simulink model "final_4"  (Simulink 7.3)
(part 2 of 2)

      |       Name		      "PQ2"
      |       Ports		      [2, 1]
      |       Position		      [1580, 1176, 1605, 1209]
      |       NamePlacement	      "alternate"
      |       DialogController	      "POWERSYS.PowerSysDialog"
      |       FontName		      "Verdana"
      |       FontSize		      11
      |       SourceBlock	      "powerlib_extras/Measurements/3-phase \nInstantaneous \nActive & Reactive Power"
      |       SourceType	      "3-phase instantaneous active and reactive power"
      |       ShowPortLabels	      "FromPortIcon"
      |       SystemSampleTime	      "-1"
      |       FunctionWithSeparateData off
      |       RTWMemSecFuncInitTerm   "Inherit from model"
      |       RTWMemSecFuncExecute    "Inherit from model"
      |       RTWMemSecDataConstants  "Inherit from model"
      |       RTWMemSecDataInternal   "Inherit from model"
      |       RTWMemSecDataParameters "Inherit from model"
      |     }
      |     Block {
      |       BlockType		      Reference
      |       Name		      "PQ3"
      |       Ports		      [2, 1]
      |       Position		      [285, 610, 325, 645]
      |       BlockMirror	      on
      |       NamePlacement	      "alternate"
      |       DialogController	      "POWERSYS.PowerSysDialog"
      |       FontName		      "Verdana"
      |       FontSize		      11
      |       SourceBlock	      "powerlib_extras/Measurements/3-phase \nInstantaneous \nActive & Reactive Power"
      |       SourceType	      "3-phase instantaneous active and reactive power"
      |       ShowPortLabels	      "FromPortIcon"
      |       SystemSampleTime	      "-1"
      |       FunctionWithSeparateData off
      |       RTWMemSecFuncInitTerm   "Inherit from model"
      |       RTWMemSecFuncExecute    "Inherit from model"
      |       RTWMemSecDataConstants  "Inherit from model"
      |       RTWMemSecDataInternal   "Inherit from model"
      |       RTWMemSecDataParameters "Inherit from model"
      |     }
      |     Block {
      |       BlockType		      Reference
      |       Name		      "PQ4"
      |       Ports		      [2, 1]
      |       Position		      [710, 561, 735, 594]
      |       NamePlacement	      "alternate"
      |       DialogController	      "POWERSYS.PowerSysDialog"
      |       FontName		      "Verdana"
      |       FontSize		      11
      |       SourceBlock	      "powerlib_extras/Measurements/3-phase \nInstantaneous \nActive & Reactive Power"
      |       SourceType	      "3-phase instantaneous active and reactive power"
      |       ShowPortLabels	      "FromPortIcon"
      |       SystemSampleTime	      "-1"
      |       FunctionWithSeparateData off
      |       RTWMemSecFuncInitTerm   "Inherit from model"
      |       RTWMemSecFuncExecute    "Inherit from model"
      |       RTWMemSecDataConstants  "Inherit from model"
      |       RTWMemSecDataInternal   "Inherit from model"
      |       RTWMemSecDataParameters "Inherit from model"
      |     }
      |     Block {
      |       BlockType		      Reference
      |       Name		      "PQ6"
      |       Ports		      [2, 1]
      |       Position		      [265, 260, 305, 295]
      |       BlockMirror	      on
      |       NamePlacement	      "alternate"
      |       DialogController	      "POWERSYS.PowerSysDialog"
      |       FontName		      "Verdana"
      |       FontSize		      11
      |       SourceBlock	      "powerlib_extras/Measurements/3-phase \nInstantaneous \nActive & Reactive Power"
      |       SourceType	      "3-phase instantaneous active and reactive power"
      |       ShowPortLabels	      "FromPortIcon"
      |       SystemSampleTime	      "-1"
      |       FunctionWithSeparateData off
      |       RTWMemSecFuncInitTerm   "Inherit from model"
      |       RTWMemSecFuncExecute    "Inherit from model"
      |       RTWMemSecDataConstants  "Inherit from model"
      |       RTWMemSecDataInternal   "Inherit from model"
      |       RTWMemSecDataParameters "Inherit from model"
      |     }
      |     Block {
      |       BlockType		      Reference
      |       Name		      "PQ7"
      |       Ports		      [2, 1]
      |       Position		      [690, 211, 715, 244]
      |       NamePlacement	      "alternate"
      |       DialogController	      "POWERSYS.PowerSysDialog"
      |       FontName		      "Verdana"
      |       FontSize		      11
      |       SourceBlock	      "powerlib_extras/Measurements/3-phase \nInstantaneous \nActive & Reactive Power"
      |       SourceType	      "3-phase instantaneous active and reactive power"
      |       ShowPortLabels	      "FromPortIcon"
      |       SystemSampleTime	      "-1"
      |       FunctionWithSeparateData off
      |       RTWMemSecFuncInitTerm   "Inherit from model"
      |       RTWMemSecFuncExecute    "Inherit from model"
      |       RTWMemSecDataConstants  "Inherit from model"
      |       RTWMemSecDataInternal   "Inherit from model"
      |       RTWMemSecDataParameters "Inherit from model"
      |     }
      |     Block {
      |       BlockType		      Reference
      |       Name		      "PQ8"
      |       Ports		      [2, 1]
      |       Position		      [710, 1126, 735, 1159]
      |       NamePlacement	      "alternate"
      |       DialogController	      "POWERSYS.PowerSysDialog"
      |       FontName		      "Verdana"
      |       FontSize		      11
      |       SourceBlock	      "powerlib_extras/Measurements/3-phase \nInstantaneous \nActive & Reactive Power"
      |       SourceType	      "3-phase instantaneous active and reactive power"
      |       ShowPortLabels	      "FromPortIcon"
      |       SystemSampleTime	      "-1"
      |       FunctionWithSeparateData off
      |       RTWMemSecFuncInitTerm   "Inherit from model"
      |       RTWMemSecFuncExecute    "Inherit from model"
      |       RTWMemSecDataConstants  "Inherit from model"
      |       RTWMemSecDataInternal   "Inherit from model"
      |       RTWMemSecDataParameters "Inherit from model"
      |     }
      |     Block {
      |       BlockType		      Reference
      |       Name		      "PQ9"
      |       Ports		      [2, 1]
      |       Position		      [1225, 215, 1265, 250]
      |       BlockMirror	      on
      |       NamePlacement	      "alternate"
      |       DialogController	      "POWERSYS.PowerSysDialog"
      |       FontName		      "Verdana"
      |       FontSize		      11
      |       SourceBlock	      "powerlib_extras/Measurements/3-phase \nInstantaneous \nActive & Reactive Power"
      |       SourceType	      "3-phase instantaneous active and reactive power"
      |       ShowPortLabels	      "FromPortIcon"
      |       SystemSampleTime	      "-1"
      |       FunctionWithSeparateData off
      |       RTWMemSecFuncInitTerm   "Inherit from model"
      |       RTWMemSecFuncExecute    "Inherit from model"
      |       RTWMemSecDataConstants  "Inherit from model"
      |       RTWMemSecDataInternal   "Inherit from model"
      |       RTWMemSecDataParameters "Inherit from model"
      |     }
      |     Block {
      |       BlockType		      Scope
      |       Name		      "PQL2"
      |       Ports		      [1]
      |       Position		      [285, 1114, 315, 1146]
      |       Floating		      off
      |       Location		      [216, 92, 540, 331]
      |       Open		      off
      |       NumInputPorts	      "1"
      |       ZoomMode		      "yonly"
      |       List {
      | 	ListType		AxesTitles
      | 	axes1			"%<SignalLabel>"
      |       }
      |       TimeRange		      "0.2"
      |       YMin		      "-2e+008"
      |       YMax		      "9e+008"
      |       SaveName		      "ScopeData25"
      |       DataFormat	      "StructureWithTime"
      |       LimitDataPoints	      off
      |       SampleTime	      "0"
      |     }
      |     Block {
      |       BlockType		      Scope
      |       Name		      "PQL4"
      |       Ports		      [1]
      |       Position		      [265, 199, 295, 231]
      |       Floating		      off
      |       Location		      [216, 92, 540, 331]
      |       Open		      off
      |       NumInputPorts	      "1"
      |       ZoomMode		      "yonly"
      |       List {
      | 	ListType		AxesTitles
      | 	axes1			"%<SignalLabel>"
      |       }
      |       TimeRange		      "0.2"
      |       YMin		      "-2e+008"
      |       YMax		      "9e+008"
      |       SaveName		      "ScopeData29"
      |       DataFormat	      "StructureWithTime"
      |       LimitDataPoints	      off
      |       SampleTime	      "0"
      |     }
      |     Block {
      |       BlockType		      Scope
      |       Name		      "PQ_L2"
      |       Ports		      [1]
      |       Position		      [285, 549, 315, 581]
      |       Floating		      off
      |       Location		      [216, 92, 540, 331]
      |       Open		      off
      |       NumInputPorts	      "1"
      |       ZoomMode		      "yonly"
      |       List {
      | 	ListType		AxesTitles
      | 	axes1			"%<SignalLabel>"
      |       }
      |       TimeRange		      "0.2"
      |       YMin		      "-2e+008"
      |       YMax		      "9e+008"
      |       SaveName		      "ScopeData14"
      |       DataFormat	      "StructureWithTime"
      |       LimitDataPoints	      off
      |       SampleTime	      "0"
      |     }
      |     Block {
      |       BlockType		      Reference
      |       Name		      "PQ_L3"
      |       Ports		      [2, 1]
      |       Position		      [285, 1175, 325, 1210]
      |       BlockMirror	      on
      |       NamePlacement	      "alternate"
      |       DialogController	      "POWERSYS.PowerSysDialog"
      |       FontName		      "Verdana"
      |       FontSize		      11
      |       SourceBlock	      "powerlib_extras/Measurements/3-phase \nInstantaneous \nActive & Reactive Power"
      |       SourceType	      "3-phase instantaneous active and reactive power"
      |       ShowPortLabels	      "FromPortIcon"
      |       SystemSampleTime	      "-1"
      |       FunctionWithSeparateData off
      |       RTWMemSecFuncInitTerm   "Inherit from model"
      |       RTWMemSecFuncExecute    "Inherit from model"
      |       RTWMemSecDataConstants  "Inherit from model"
      |       RTWMemSecDataInternal   "Inherit from model"
      |       RTWMemSecDataParameters "Inherit from model"
      |     }
      |     Block {
      |       BlockType		      Scope
      |       Name		      "PQ_L4"
      |       Ports		      [1]
      |       Position		      [1225, 154, 1255, 186]
      |       Floating		      off
      |       Location		      [216, 92, 540, 331]
      |       Open		      off
      |       NumInputPorts	      "1"
      |       ZoomMode		      "yonly"
      |       List {
      | 	ListType		AxesTitles
      | 	axes1			"%<SignalLabel>"
      |       }
      |       TimeRange		      "0.2"
      |       YMin		      "-2e+008"
      |       YMax		      "9e+008"
      |       SaveName		      "ScopeData47"
      |       DataFormat	      "StructureWithTime"
      |       LimitDataPoints	      off
      |       SampleTime	      "0"
      |     }
      |     Block {
      |       BlockType		      Scope
      |       Name		      "PQ_L5"
      |       Ports		      [1]
      |       Position		      [1155, 1164, 1185, 1196]
      |       Floating		      off
      |       Location		      [216, 92, 540, 331]
      |       Open		      off
      |       NumInputPorts	      "1"
      |       ZoomMode		      "yonly"
      |       List {
      | 	ListType		AxesTitles
      | 	axes1			"%<SignalLabel>"
      |       }
      |       TimeRange		      "0.2"
      |       YMin		      "-2e+008"
      |       YMax		      "9e+008"
      |       SaveName		      "ScopeData4"
      |       DataFormat	      "StructureWithTime"
      |       LimitDataPoints	      off
      |       SampleTime	      "0"
      |     }
      |     Block {
      |       BlockType		      Scope
      |       Name		      "PQs_1"
      |       Ports		      [1]
      |       Position		      [715, 252, 740, 278]
      |       Floating		      off
      |       Location		      [784, 486, 1108, 725]
      |       Open		      off
      |       NumInputPorts	      "1"
      |       ZoomMode		      "yonly"
      |       List {
      | 	ListType		AxesTitles
      | 	axes1			"%<SignalLabel>"
      |       }
      |       TimeRange		      "0.25"
      |       YMin		      "-250"
      |       YMax		      "4000"
      |       SaveName		      "ScopeData30"
      |       DataFormat	      "StructureWithTime"
      |       LimitDataPoints	      off
      |       SampleTime	      "0"
      |     }
      |     Block {
      |       BlockType		      Scope
      |       Name		      "PQs_2"
      |       Ports		      [1]
      |       Position		      [735, 602, 760, 628]
      |       Floating		      off
      |       Location		      [784, 486, 1108, 725]
      |       Open		      off
      |       NumInputPorts	      "1"
      |       ZoomMode		      "yonly"
      |       List {
      | 	ListType		AxesTitles
      | 	axes1			"%<SignalLabel>"
      |       }
      |       TimeRange		      "0.25"
      |       YMin		      "-250"
      |       YMax		      "4000"
      |       SaveName		      "ScopeData15"
      |       DataFormat	      "StructureWithTime"
      |       LimitDataPoints	      off
      |       SampleTime	      "0"
      |     }
      |     Block {
      |       BlockType		      Scope
      |       Name		      "PQs_3"
      |       Ports		      [1]
      |       Position		      [735, 1167, 760, 1193]
      |       Floating		      off
      |       Location		      [784, 486, 1108, 725]
      |       Open		      off
      |       NumInputPorts	      "1"
      |       ZoomMode		      "yonly"
      |       List {
      | 	ListType		AxesTitles
      | 	axes1			"%<SignalLabel>"
      |       }
      |       TimeRange		      "0.25"
      |       YMin		      "-250"
      |       YMax		      "4000"
      |       SaveName		      "ScopeData26"
      |       DataFormat	      "StructureWithTime"
      |       LimitDataPoints	      off
      |       SampleTime	      "0"
      |     }
      |     Block {
      |       BlockType		      Scope
      |       Name		      "PQs_4"
      |       Ports		      [1]
      |       Position		      [1675, 207, 1700, 233]
      |       Floating		      off
      |       Location		      [784, 486, 1108, 725]
      |       Open		      off
      |       NumInputPorts	      "1"
      |       ZoomMode		      "yonly"
      |       List {
      | 	ListType		AxesTitles
      | 	axes1			"%<SignalLabel>"
      |       }
      |       TimeRange		      "0.25"
      |       YMin		      "-250"
      |       YMax		      "4000"
      |       SaveName		      "ScopeData48"
      |       DataFormat	      "StructureWithTime"
      |       LimitDataPoints	      off
      |       SampleTime	      "0"
      |     }
      |     Block {
      |       BlockType		      Scope
      |       Name		      "PQs_5"
      |       Ports		      [1]
      |       Position		      [1605, 1217, 1630, 1243]
      |       Floating		      off
      |       Location		      [784, 486, 1108, 725]
      |       Open		      off
      |       NumInputPorts	      "1"
      |       ZoomMode		      "yonly"
      |       List {
      | 	ListType		AxesTitles
      | 	axes1			"%<SignalLabel>"
      |       }
      |       TimeRange		      "0.25"
      |       YMin		      "-250"
      |       YMax		      "4000"
      |       SaveName		      "ScopeData5"
      |       DataFormat	      "StructureWithTime"
      |       LimitDataPoints	      off
      |       SampleTime	      "0"
      |     }
      |     Block {
      |       BlockType		      Reference
      |       Name		      "RMS1"
      |       Ports		      [1, 1]
      |       Position		      [1635, 1248, 1655, 1282]
      |       DialogController	      "POWERSYS.PowerSysDialog"
      |       FontName		      "Verdana"
      |       FontSize		      11
      |       SourceBlock	      "powerlib_extras/Measurements/RMS"
      |       SourceType	      "RMS"
      |       ShowPortLabels	      "FromPortIcon"
      |       SystemSampleTime	      "-1"
      |       FunctionWithSeparateData off
      |       RTWMemSecFuncInitTerm   "Inherit from model"
      |       RTWMemSecFuncExecute    "Inherit from model"
      |       RTWMemSecDataConstants  "Inherit from model"
      |       RTWMemSecDataInternal   "Inherit from model"
      |       RTWMemSecDataParameters "Inherit from model"
      |       f1		      "50"
      |     }
      |     Block {
      |       BlockType		      Reference
      |       Name		      "RMS10"
      |       Ports		      [1, 1]
      |       Position		      [1705, 169, 1725, 201]
      |       DialogController	      "POWERSYS.PowerSysDialog"
      |       FontName		      "Verdana"
      |       FontSize		      11
      |       SourceBlock	      "powerlib_extras/Measurements/RMS"
      |       SourceType	      "RMS"
      |       ShowPortLabels	      "FromPortIcon"
      |       SystemSampleTime	      "-1"
      |       FunctionWithSeparateData off
      |       RTWMemSecFuncInitTerm   "Inherit from model"
      |       RTWMemSecFuncExecute    "Inherit from model"
      |       RTWMemSecDataConstants  "Inherit from model"
      |       RTWMemSecDataInternal   "Inherit from model"
      |       RTWMemSecDataParameters "Inherit from model"
      |       f1		      "50"
      |     }
      |     Block {
      |       BlockType		      Reference
      |       Name		      "RMS2"
      |       Ports		      [1, 1]
      |       Position		      [1635, 1179, 1655, 1211]
      |       DialogController	      "POWERSYS.PowerSysDialog"
      |       FontName		      "Verdana"
      |       FontSize		      11
      |       SourceBlock	      "powerlib_extras/Measurements/RMS"
      |       SourceType	      "RMS"
      |       ShowPortLabels	      "FromPortIcon"
      |       SystemSampleTime	      "-1"
      |       FunctionWithSeparateData off
      |       RTWMemSecFuncInitTerm   "Inherit from model"
      |       RTWMemSecFuncExecute    "Inherit from model"
      |       RTWMemSecDataConstants  "Inherit from model"
      |       RTWMemSecDataInternal   "Inherit from model"
      |       RTWMemSecDataParameters "Inherit from model"
      |       f1		      "50"
      |     }
      |     Block {
      |       BlockType		      Reference
      |       Name		      "RMS3"
      |       Ports		      [1, 1]
      |       Position		      [765, 633, 785, 667]
      |       DialogController	      "POWERSYS.PowerSysDialog"
      |       FontName		      "Verdana"
      |       FontSize		      11
      |       SourceBlock	      "powerlib_extras/Measurements/RMS"
      |       SourceType	      "RMS"
      |       ShowPortLabels	      "FromPortIcon"
      |       SystemSampleTime	      "-1"
      |       FunctionWithSeparateData off
      |       RTWMemSecFuncInitTerm   "Inherit from model"
      |       RTWMemSecFuncExecute    "Inherit from model"
      |       RTWMemSecDataConstants  "Inherit from model"
      |       RTWMemSecDataInternal   "Inherit from model"
      |       RTWMemSecDataParameters "Inherit from model"
      |       f1		      "50"
      |     }
      |     Block {
      |       BlockType		      Reference
      |       Name		      "RMS4"
      |       Ports		      [1, 1]
      |       Position		      [765, 1198, 785, 1232]
      |       DialogController	      "POWERSYS.PowerSysDialog"
      |       FontName		      "Verdana"
      |       FontSize		      11
      |       SourceBlock	      "powerlib_extras/Measurements/RMS"
      |       SourceType	      "RMS"
      |       ShowPortLabels	      "FromPortIcon"
      |       SystemSampleTime	      "-1"
      |       FunctionWithSeparateData off
      |       RTWMemSecFuncInitTerm   "Inherit from model"
      |       RTWMemSecFuncExecute    "Inherit from model"
      |       RTWMemSecDataConstants  "Inherit from model"
      |       RTWMemSecDataInternal   "Inherit from model"
      |       RTWMemSecDataParameters "Inherit from model"
      |       f1		      "50"
      |     }
      |     Block {
      |       BlockType		      Reference
      |       Name		      "RMS5"
      |       Ports		      [1, 1]
      |       Position		      [765, 1129, 785, 1161]
      |       DialogController	      "POWERSYS.PowerSysDialog"
      |       FontName		      "Verdana"
      |       FontSize		      11
      |       SourceBlock	      "powerlib_extras/Measurements/RMS"
      |       SourceType	      "RMS"
      |       ShowPortLabels	      "FromPortIcon"
      |       SystemSampleTime	      "-1"
      |       FunctionWithSeparateData off
      |       RTWMemSecFuncInitTerm   "Inherit from model"
      |       RTWMemSecFuncExecute    "Inherit from model"
      |       RTWMemSecDataConstants  "Inherit from model"
      |       RTWMemSecDataInternal   "Inherit from model"
      |       RTWMemSecDataParameters "Inherit from model"
      |       f1		      "50"
      |     }
      |     Block {
      |       BlockType		      Reference
      |       Name		      "RMS6"
      |       Ports		      [1, 1]
      |       Position		      [760, 564, 780, 596]
      |       DialogController	      "POWERSYS.PowerSysDialog"
      |       FontName		      "Verdana"
      |       FontSize		      11
      |       SourceBlock	      "powerlib_extras/Measurements/RMS"
      |       SourceType	      "RMS"
      |       ShowPortLabels	      "FromPortIcon"
      |       SystemSampleTime	      "-1"
      |       FunctionWithSeparateData off
      |       RTWMemSecFuncInitTerm   "Inherit from model"
      |       RTWMemSecFuncExecute    "Inherit from model"
      |       RTWMemSecDataConstants  "Inherit from model"
      |       RTWMemSecDataInternal   "Inherit from model"
      |       RTWMemSecDataParameters "Inherit from model"
      |       f1		      "50"
      |     }
      |     Block {
      |       BlockType		      Reference
      |       Name		      "RMS7"
      |       Ports		      [1, 1]
      |       Position		      [745, 283, 765, 317]
      |       DialogController	      "POWERSYS.PowerSysDialog"
      |       FontName		      "Verdana"
      |       FontSize		      11
      |       SourceBlock	      "powerlib_extras/Measurements/RMS"
      |       SourceType	      "RMS"
      |       ShowPortLabels	      "FromPortIcon"
      |       SystemSampleTime	      "-1"
      |       FunctionWithSeparateData off
      |       RTWMemSecFuncInitTerm   "Inherit from model"
      |       RTWMemSecFuncExecute    "Inherit from model"
      |       RTWMemSecDataConstants  "Inherit from model"
      |       RTWMemSecDataInternal   "Inherit from model"
      |       RTWMemSecDataParameters "Inherit from model"
      |       f1		      "50"
      |     }
      |     Block {
      |       BlockType		      Reference
      |       Name		      "RMS8"
      |       Ports		      [1, 1]
      |       Position		      [745, 214, 765, 246]
      |       DialogController	      "POWERSYS.PowerSysDialog"
      |       FontName		      "Verdana"
      |       FontSize		      11
      |       SourceBlock	      "powerlib_extras/Measurements/RMS"
      |       SourceType	      "RMS"
      |       ShowPortLabels	      "FromPortIcon"
      |       SystemSampleTime	      "-1"
      |       FunctionWithSeparateData off
      |       RTWMemSecFuncInitTerm   "Inherit from model"
      |       RTWMemSecFuncExecute    "Inherit from model"
      |       RTWMemSecDataConstants  "Inherit from model"
      |       RTWMemSecDataInternal   "Inherit from model"
      |       RTWMemSecDataParameters "Inherit from model"
      |       f1		      "50"
      |     }
      |     Block {
      |       BlockType		      Reference
      |       Name		      "RMS9"
      |       Ports		      [1, 1]
      |       Position		      [1705, 238, 1725, 272]
      |       DialogController	      "POWERSYS.PowerSysDialog"
      |       FontName		      "Verdana"
      |       FontSize		      11
      |       SourceBlock	      "powerlib_extras/Measurements/RMS"
      |       SourceType	      "RMS"
      |       ShowPortLabels	      "FromPortIcon"
      |       SystemSampleTime	      "-1"
      |       FunctionWithSeparateData off
      |       RTWMemSecFuncInitTerm   "Inherit from model"
      |       RTWMemSecFuncExecute    "Inherit from model"
      |       RTWMemSecDataConstants  "Inherit from model"
      |       RTWMemSecDataInternal   "Inherit from model"
      |       RTWMemSecDataParameters "Inherit from model"
      |       f1		      "50"
      |     }
      |     Block {
      |       BlockType		      SubSystem
      |       Name		      "Subsystem1"
      |       Ports		      [3, 1]
      |       Position		      [930, 1232, 970, 1328]
      |       BlockMirror	      on
      |       NamePlacement	      "alternate"
      |       MinAlgLoopOccurrences   off
      |       PropExecContextOutsideSubsystem off
      |       RTWSystemCode	      "Auto"
      |       FunctionWithSeparateData off
      |       Opaque		      off
      |       RequestExecContextInheritance off
      |       MaskHideContents	      off
      |       System {
      | 	Name			"Subsystem1"
      | 	Location		[4, 82, 1272, 776]
      | 	Open			off
      | 	ModelBrowserVisibility	off
      | 	ModelBrowserWidth	200
      | 	ScreenColor		"white"
      | 	PaperOrientation	"landscape"
      | 	PaperPositionMode	"auto"
      | 	PaperType		"usletter"
      | 	PaperUnits		"inches"
      | 	TiledPaperMargins	[0.500000, 0.500000, 0.500000, 0.500000]
      | 	TiledPageScale		1
      | 	ShowPageBoundaries	off
      | 	ZoomFactor		"100"
      | 	Block {
      | 	  BlockType		  Inport
      | 	  Name			  "PL"
      | 	  Position		  [185, 373, 215, 387]
      | 	  IconDisplay		  "Port number"
      | 	  OutDataType		  "fixdt(1, 16)"
      | 	  OutScaling		  "2^0"
      | 	}
      | 	Block {
      | 	  BlockType		  Inport
      | 	  Name			  "iL"
      | 	  Position		  [185, 133, 215, 147]
      | 	  Port			  "2"
      | 	  IconDisplay		  "Port number"
      | 	  OutDataType		  "fixdt(1, 16)"
      | 	  OutScaling		  "2^0"
      | 	}
      | 	Block {
      | 	  BlockType		  Inport
      | 	  Name			  "vL"
      | 	  Position		  [185, 258, 215, 272]
      | 	  Port			  "3"
      | 	  IconDisplay		  "Port number"
      | 	  OutDataType		  "fixdt(1, 16)"
      | 	  OutScaling		  "2^0"
      | 	}
      | 	Block {
      | 	  BlockType		  SubSystem
      | 	  Name			  "1 constant power"
      | 	  Ports			  [1, 1]
      | 	  Position		  [690, 124, 790, 166]
      | 	  MinAlgLoopOccurrences	  off
      | 	  PropExecContextOutsideSubsystem off
      | 	  RTWSystemCode		  "Auto"
      | 	  FunctionWithSeparateData off
      | 	  Opaque		  off
      | 	  RequestExecContextInheritance	off
      | 	  MaskHideContents	  off
      | 	  System {
      | 	    Name		    "1 constant power"
      | 	    Location		    [2, 82, 1270, 754]
      | 	    Open		    off
      | 	    ModelBrowserVisibility  off
      | 	    ModelBrowserWidth	    200
      | 	    ScreenColor		    "white"
      | 	    PaperOrientation	    "landscape"
      | 	    PaperPositionMode	    "auto"
      | 	    PaperType		    "usletter"
      | 	    PaperUnits		    "inches"
      | 	    TiledPaperMargins	    [0.500000, 0.500000, 0.500000, 0.500000]
      | 	    TiledPageScale	    1
      | 	    ShowPageBoundaries	    off
      | 	    ZoomFactor		    "100"
      | 	    Block {
      | 	      BlockType		      Inport
      | 	      Name		      "In1"
      | 	      Position		      [120, 313, 150, 327]
      | 	      IconDisplay	      "Port number"
      | 	      OutDataType	      "fixdt(1, 16)"
      | 	      OutScaling	      "2^0"
      | 	    }
      | 	    Block {
      | 	      BlockType		      Demux
      | 	      Name		      "Demux"
      | 	      Ports		      [1, 3]
      | 	      Position		      [1010, 406, 1015, 444]
      | 	      ShowName		      off
      | 	      Outputs		      "3"
      | 	      DisplayOption	      "bar"
      | 	    }
      | 	    Block {
      | 	      BlockType		      Demux
      | 	      Name		      "Demux1"
      | 	      Ports		      [1, 7]
      | 	      Position		      [185, 248, 190, 392]
      | 	      ShowName		      off
      | 	      Outputs		      "7"
      | 	      DisplayOption	      "bar"
      | 	    }
      | 	    Block {
      | 	      BlockType		      Reference
      | 	      Name		      "Discrete \nMean value"
      | 	      Ports		      [1, 1]
      | 	      Position		      [375, 406, 435, 464]
      | 	      DialogController	      "POWERSYS.PowerSysDialog"
      | 	      SourceBlock	      "powerlib_extras/Discrete\nMeasurements/Discrete \nMean value"
      | 	      SourceType	      "Discrete Mean value"
      | 	      ShowPortLabels	      "FromPortIcon"
      | 	      SystemSampleTime	      "-1"
      | 	      FunctionWithSeparateData off
      | 	      RTWMemSecFuncInitTerm   "Inherit from model"
      | 	      RTWMemSecFuncExecute    "Inherit from model"
      | 	      RTWMemSecDataConstants  "Inherit from model"
      | 	      RTWMemSecDataInternal   "Inherit from model"
      | 	      RTWMemSecDataParameters "Inherit from model"
      | 	      Freq		      "50"
      | 	      Vinit		      ".001"
      | 	      Ts		      "50e-6"
      | 	    }
      | 	    Block {
      | 	      BlockType		      SubSystem
      | 	      Name		      "Embedded\nMATLAB Function"
      | 	      Ports		      [1, 1]
      | 	      Position		      [370, 257, 440, 303]
      | 	      NamePlacement	      "alternate"
      | 	      PermitHierarchicalResolution "ExplicitOnly"
      | 	      TreatAsAtomicUnit	      on
      | 	      MinAlgLoopOccurrences   off
      | 	      PropExecContextOutsideSubsystem off
      | 	      RTWSystemCode	      "Auto"
      | 	      FunctionWithSeparateData off
      | 	      Opaque		      off
      | 	      Array {
      | 		Type			"Handle"
      | 		Dimension		0
      | 		PropName		"AvailSigsLoadSave"
      | 	      }
      | 	      RequestExecContextInheritance off
      | 	      MaskHideContents	      off
      | 	      MaskType		      "Stateflow"
      | 	      MaskDescription	      "Embedded MATLAB block"
      | 	      MaskDisplay	      "disp('fcn');"
      | 	      MaskSelfModifiable      on
      | 	      MaskIconFrame	      on
      | 	      MaskIconOpaque	      off
      | 	      MaskIconRotate	      "none"
      | 	      MaskPortRotate	      "default"
      | 	      MaskIconUnits	      "autoscale"
      | 	      System {
      | 		Name			"Embedded\nMATLAB Function"
      | 		Location		[257, 457, 812, 717]
      | 		Open			off
      | 		ModelBrowserVisibility	off
      | 		ModelBrowserWidth	200
      | 		ScreenColor		"white"
      | 		PaperOrientation	"landscape"
      | 		PaperPositionMode	"auto"
      | 		PaperType		"usletter"
      | 		PaperUnits		"inches"
      | 		TiledPaperMargins	[0.500000, 0.500000, 0.500000, 0.500000]
      | 		TiledPageScale		1
      | 		ShowPageBoundaries	off
      | 		ZoomFactor		"100"
      | 		Block {
      | 		  BlockType		  Inport
      | 		  Name			  "a"
      | 		  Position		  [20, 101, 40, 119]
      | 		  IconDisplay		  "Port number"
      | 		  OutDataType		  "sfix(16)"
      | 		  OutScaling		  "2^0"
      | 		}
      | 		Block {
      | 		  BlockType		  Demux
      | 		  Name			  " Demux "
      | 		  Ports			  [1, 1]
      | 		  Position		  [270, 160, 320, 200]
      | 		  Outputs		  "1"
      | 		}
      | 		Block {
      | 		  BlockType		  "S-Function"
      | 		  Name			  " SFunction "
      | 		  Tag			  "Stateflow S-Function final_4 3"
      | 		  Ports			  [1, 2]
      | 		  Position		  [180, 100, 230, 160]
      | 		  FunctionName		  "sf_sfun"
      | 		  PortCounts		  "[1 2]"
      | 		  EnableBusSupport	  on
      | 		  Port {
      | 		    PortNumber		    2
      | 		    Name		    "y"
      | 		    RTWStorageClass	    "Auto"
      | 		    DataLoggingNameMode	    "SignalName"
      | 		  }
      | 		}
      | 		Block {
      | 		  BlockType		  Terminator
      | 		  Name			  " Terminator "
      | 		  Position		  [460, 171, 480, 189]
      | 		}
      | 		Block {
      | 		  BlockType		  Outport
      | 		  Name			  "y"
      | 		  Position		  [460, 101, 480, 119]
      | 		  IconDisplay		  "Port number"
      | 		  OutDataType		  "sfix(16)"
      | 		  OutScaling		  "2^0"
      | 		}
      | 		Line {
      | 		  SrcBlock		  " Demux "
      | 		  SrcPort		  1
      | 		  DstBlock		  " Terminator "
      | 		  DstPort		  1
      | 		}
      | 		Line {
      | 		  Name			  "y"
      | 		  Labels		  [0, 0]
      | 		  SrcBlock		  " SFunction "
      | 		  SrcPort		  2
      | 		  DstBlock		  "y"
      | 		  DstPort		  1
      | 		}
      | 		Line {
      | 		  SrcBlock		  "a"
      | 		  SrcPort		  1
      | 		  DstBlock		  " SFunction "
      | 		  DstPort		  1
      | 		}
      | 		Line {
      | 		  SrcBlock		  " SFunction "
      | 		  SrcPort		  1
      | 		  DstBlock		  " Demux "
      | 		  DstPort		  1
      | 		}
      | 	      }
      | 	    }
      | 	    Block {
      | 	      BlockType		      SubSystem
      | 	      Name		      "Embedded\nMATLAB Function1"
      | 	      Ports		      [1, 1]
      | 	      Position		      [370, 317, 440, 363]
      | 	      PermitHierarchicalResolution "ExplicitOnly"
      | 	      TreatAsAtomicUnit	      on
      | 	      MinAlgLoopOccurrences   off
      | 	      PropExecContextOutsideSubsystem off
      | 	      RTWSystemCode	      "Auto"
      | 	      FunctionWithSeparateData off
      | 	      Opaque		      off
      | 	      Array {
      | 		Type			"Handle"
      | 		Dimension		0
      | 		PropName		"AvailSigsLoadSave"
      | 	      }
      | 	      RequestExecContextInheritance off
      | 	      MaskHideContents	      off
      | 	      MaskType		      "Stateflow"
      | 	      MaskDescription	      "Embedded MATLAB block"
      | 	      MaskDisplay	      "disp('fcn');"
      | 	      MaskSelfModifiable      on
      | 	      MaskIconFrame	      on
      | 	      MaskIconOpaque	      off
      | 	      MaskIconRotate	      "none"
      | 	      MaskPortRotate	      "default"
      | 	      MaskIconUnits	      "autoscale"
      | 	      System {
      | 		Name			"Embedded\nMATLAB Function1"
      | 		Location		[257, 457, 812, 717]
      | 		Open			off
      | 		ModelBrowserVisibility	off
      | 		ModelBrowserWidth	200
      | 		ScreenColor		"white"
      | 		PaperOrientation	"landscape"
      | 		PaperPositionMode	"auto"
      | 		PaperType		"usletter"
      | 		PaperUnits		"inches"
      | 		TiledPaperMargins	[0.500000, 0.500000, 0.500000, 0.500000]
      | 		TiledPageScale		1
      | 		ShowPageBoundaries	off
      | 		ZoomFactor		"100"
      | 		Block {
      | 		  BlockType		  Inport
      | 		  Name			  "b"
      | 		  Position		  [20, 101, 40, 119]
      | 		  IconDisplay		  "Port number"
      | 		  OutDataType		  "sfix(16)"
      | 		  OutScaling		  "2^0"
      | 		}
      | 		Block {
      | 		  BlockType		  Demux
      | 		  Name			  " Demux "
      | 		  Ports			  [1, 1]
      | 		  Position		  [270, 160, 320, 200]
      | 		  Outputs		  "1"
      | 		}
      | 		Block {
      | 		  BlockType		  "S-Function"
      | 		  Name			  " SFunction "
      | 		  Tag			  "Stateflow S-Function final_4 4"
      | 		  Ports			  [1, 2]
      | 		  Position		  [180, 100, 230, 160]
      | 		  FunctionName		  "sf_sfun"
      | 		  PortCounts		  "[1 2]"
      | 		  EnableBusSupport	  on
      | 		  Port {
      | 		    PortNumber		    2
      | 		    Name		    "y"
      | 		    RTWStorageClass	    "Auto"
      | 		    DataLoggingNameMode	    "SignalName"
      | 		  }
      | 		}
      | 		Block {
      | 		  BlockType		  Terminator
      | 		  Name			  " Terminator "
      | 		  Position		  [460, 171, 480, 189]
      | 		}
      | 		Block {
      | 		  BlockType		  Outport
      | 		  Name			  "y"
      | 		  Position		  [460, 101, 480, 119]
      | 		  IconDisplay		  "Port number"
      | 		  OutDataType		  "sfix(16)"
      | 		  OutScaling		  "2^0"
      | 		}
      | 		Line {
      | 		  SrcBlock		  " Demux "
      | 		  SrcPort		  1
      | 		  DstBlock		  " Terminator "
      | 		  DstPort		  1
      | 		}
      | 		Line {
      | 		  Name			  "y"
      | 		  Labels		  [0, 0]
      | 		  SrcBlock		  " SFunction "
      | 		  SrcPort		  2
      | 		  DstBlock		  "y"
      | 		  DstPort		  1
      | 		}
      | 		Line {
      | 		  SrcBlock		  "b"
      | 		  SrcPort		  1
      | 		  DstBlock		  " SFunction "
      | 		  DstPort		  1
      | 		}
      | 		Line {
      | 		  SrcBlock		  " SFunction "
      | 		  SrcPort		  1
      | 		  DstBlock		  " Demux "
      | 		  DstPort		  1
      | 		}
      | 	      }
      | 	    }
      | 	    Block {
      | 	      BlockType		      SubSystem
      | 	      Name		      "Embedded\nMATLAB Function3"
      | 	      Ports		      [1, 1]
      | 	      Position		      [805, 337, 875, 383]
      | 	      PermitHierarchicalResolution "ExplicitOnly"
      | 	      TreatAsAtomicUnit	      on
      | 	      MinAlgLoopOccurrences   off
      | 	      PropExecContextOutsideSubsystem off
      | 	      RTWSystemCode	      "Auto"
      | 	      FunctionWithSeparateData off
      | 	      Opaque		      off
      | 	      Array {
      | 		Type			"Handle"
      | 		Dimension		0
      | 		PropName		"AvailSigsLoadSave"
      | 	      }
      | 	      RequestExecContextInheritance off
      | 	      MaskHideContents	      off
      | 	      MaskType		      "Stateflow"
      | 	      MaskDescription	      "Embedded MATLAB block"
      | 	      MaskDisplay	      "disp('fcn');"
      | 	      MaskSelfModifiable      on
      | 	      MaskIconFrame	      on
      | 	      MaskIconOpaque	      off
      | 	      MaskIconRotate	      "none"
      | 	      MaskPortRotate	      "default"
      | 	      MaskIconUnits	      "autoscale"
      | 	      System {
      | 		Name			"Embedded\nMATLAB Function3"
      | 		Location		[257, 457, 812, 717]
      | 		Open			off
      | 		ModelBrowserVisibility	off
      | 		ModelBrowserWidth	200
      | 		ScreenColor		"white"
      | 		PaperOrientation	"landscape"
      | 		PaperPositionMode	"auto"
      | 		PaperType		"usletter"
      | 		PaperUnits		"inches"
      | 		TiledPaperMargins	[0.500000, 0.500000, 0.500000, 0.500000]
      | 		TiledPageScale		1
      | 		ShowPageBoundaries	off
      | 		ZoomFactor		"100"
      | 		Block {
      | 		  BlockType		  Inport
      | 		  Name			  "h"
      | 		  Position		  [20, 101, 40, 119]
      | 		  IconDisplay		  "Port number"
      | 		  OutDataType		  "sfix(16)"
      | 		  OutScaling		  "2^0"
      | 		}
      | 		Block {
      | 		  BlockType		  Demux
      | 		  Name			  " Demux "
      | 		  Ports			  [1, 1]
      | 		  Position		  [270, 160, 320, 200]
      | 		  Outputs		  "1"
      | 		}
      | 		Block {
      | 		  BlockType		  "S-Function"
      | 		  Name			  " SFunction "
      | 		  Tag			  "Stateflow S-Function final_4 5"
      | 		  Ports			  [1, 2]
      | 		  Position		  [180, 100, 230, 160]
      | 		  FunctionName		  "sf_sfun"
      | 		  PortCounts		  "[1 2]"
      | 		  EnableBusSupport	  on
      | 		  Port {
      | 		    PortNumber		    2
      | 		    Name		    "y"
      | 		    RTWStorageClass	    "Auto"
      | 		    DataLoggingNameMode	    "SignalName"
      | 		  }
      | 		}
      | 		Block {
      | 		  BlockType		  Terminator
      | 		  Name			  " Terminator "
      | 		  Position		  [460, 171, 480, 189]
      | 		}
      | 		Block {
      | 		  BlockType		  Outport
      | 		  Name			  "y"
      | 		  Position		  [460, 101, 480, 119]
      | 		  IconDisplay		  "Port number"
      | 		  OutDataType		  "sfix(16)"
      | 		  OutScaling		  "2^0"
      | 		}
      | 		Line {
      | 		  SrcBlock		  " Demux "
      | 		  SrcPort		  1
      | 		  DstBlock		  " Terminator "
      | 		  DstPort		  1
      | 		}
      | 		Line {
      | 		  Name			  "y"
      | 		  Labels		  [0, 0]
      | 		  SrcBlock		  " SFunction "
      | 		  SrcPort		  2
      | 		  DstBlock		  "y"
      | 		  DstPort		  1
      | 		}
      | 		Line {
      | 		  SrcBlock		  "h"
      | 		  SrcPort		  1
      | 		  DstBlock		  " SFunction "
      | 		  DstPort		  1
      | 		}
      | 		Line {
      | 		  SrcBlock		  " SFunction "
      | 		  SrcPort		  1
      | 		  DstBlock		  " Demux "
      | 		  DstPort		  1
      | 		}
      | 	      }
      | 	    }
      | 	    Block {
      | 	      BlockType		      SubSystem
      | 	      Name		      "Embedded\nMATLAB Function4"
      | 	      Ports		      [1, 1]
      | 	      Position		      [655, 337, 725, 383]
      | 	      PermitHierarchicalResolution "ExplicitOnly"
      | 	      TreatAsAtomicUnit	      on
      | 	      MinAlgLoopOccurrences   off
      | 	      PropExecContextOutsideSubsystem off
      | 	      RTWSystemCode	      "Auto"
      | 	      FunctionWithSeparateData off
      | 	      Opaque		      off
      | 	      Array {
      | 		Type			"Handle"
      | 		Dimension		0
      | 		PropName		"AvailSigsLoadSave"
      | 	      }
      | 	      RequestExecContextInheritance off
      | 	      MaskHideContents	      off
      | 	      MaskType		      "Stateflow"
      | 	      MaskDescription	      "Embedded MATLAB block"
      | 	      MaskDisplay	      "disp('fcn');"
      | 	      MaskSelfModifiable      on
      | 	      MaskIconFrame	      on
      | 	      MaskIconOpaque	      off
      | 	      MaskIconRotate	      "none"
      | 	      MaskPortRotate	      "default"
      | 	      MaskIconUnits	      "autoscale"
      | 	      System {
      | 		Name			"Embedded\nMATLAB Function4"
      | 		Location		[257, 457, 812, 717]
      | 		Open			off
      | 		ModelBrowserVisibility	off
      | 		ModelBrowserWidth	200
      | 		ScreenColor		"white"
      | 		PaperOrientation	"landscape"
      | 		PaperPositionMode	"auto"
      | 		PaperType		"usletter"
      | 		PaperUnits		"inches"
      | 		TiledPaperMargins	[0.500000, 0.500000, 0.500000, 0.500000]
      | 		TiledPageScale		1
      | 		ShowPageBoundaries	off
      | 		ZoomFactor		"100"
      | 		Block {
      | 		  BlockType		  Inport
      | 		  Name			  "a"
      | 		  Position		  [20, 101, 40, 119]
      | 		  IconDisplay		  "Port number"
      | 		  OutDataType		  "sfix(16)"
      | 		  OutScaling		  "2^0"
      | 		}
      | 		Block {
      | 		  BlockType		  Demux
      | 		  Name			  " Demux "
      | 		  Ports			  [1, 1]
      | 		  Position		  [270, 160, 320, 200]
      | 		  Outputs		  "1"
      | 		}
      | 		Block {
      | 		  BlockType		  "S-Function"
      | 		  Name			  " SFunction "
      | 		  Tag			  "Stateflow S-Function final_4 6"
      | 		  Ports			  [1, 2]
      | 		  Position		  [180, 100, 230, 160]
      | 		  FunctionName		  "sf_sfun"
      | 		  PortCounts		  "[1 2]"
      | 		  EnableBusSupport	  on
      | 		  Port {
      | 		    PortNumber		    2
      | 		    Name		    "y"
      | 		    RTWStorageClass	    "Auto"
      | 		    DataLoggingNameMode	    "SignalName"
      | 		  }
      | 		}
      | 		Block {
      | 		  BlockType		  Terminator
      | 		  Name			  " Terminator "
      | 		  Position		  [460, 171, 480, 189]
      | 		}
      | 		Block {
      | 		  BlockType		  Outport
      | 		  Name			  "y"
      | 		  Position		  [460, 101, 480, 119]
      | 		  IconDisplay		  "Port number"
      | 		  OutDataType		  "sfix(16)"
      | 		  OutScaling		  "2^0"
      | 		}
      | 		Line {
      | 		  SrcBlock		  " Demux "
      | 		  SrcPort		  1
      | 		  DstBlock		  " Terminator "
      | 		  DstPort		  1
      | 		}
      | 		Line {
      | 		  Name			  "y"
      | 		  Labels		  [0, 0]
      | 		  SrcBlock		  " SFunction "
      | 		  SrcPort		  2
      | 		  DstBlock		  "y"
      | 		  DstPort		  1
      | 		}
      | 		Line {
      | 		  SrcBlock		  "a"
      | 		  SrcPort		  1
      | 		  DstBlock		  " SFunction "
      | 		  DstPort		  1
      | 		}
      | 		Line {
      | 		  SrcBlock		  " SFunction "
      | 		  SrcPort		  1
      | 		  DstBlock		  " Demux "
      | 		  DstPort		  1
      | 		}
      | 	      }
      | 	    }
      | 	    Block {
      | 	      BlockType		      Mux
      | 	      Name		      "Mux1"
      | 	      Ports		      [3, 1]
      | 	      Position		      [555, 328, 560, 392]
      | 	      ShowName		      off
      | 	      Inputs		      "3"
      | 	      DisplayOption	      "bar"
      | 	    }
      | 	    Block {
      | 	      BlockType		      Mux
      | 	      Name		      "Mux3"
      | 	      Ports		      [3, 1]
      | 	      Position		      [240, 247, 245, 313]
      | 	      ShowName		      off
      | 	      Inputs		      "3"
      | 	      DisplayOption	      "bar"
      | 	    }
      | 	    Block {
      | 	      BlockType		      Mux
      | 	      Name		      "Mux4"
      | 	      Ports		      [3, 1]
      | 	      Position		      [240, 307, 245, 373]
      | 	      ShowName		      off
      | 	      Inputs		      "3"
      | 	      DisplayOption	      "bar"
      | 	    }
      | 	    Block {
      | 	      BlockType		      Scope
      | 	      Name		      "Scope1"
      | 	      Ports		      [3]
      | 	      Position		      [1040, 409, 1070, 441]
      | 	      Floating		      off
      | 	      Location		      [5, 98, 1033, 741]
      | 	      Open		      off
      | 	      NumInputPorts	      "3"
      | 	      List {
      | 		ListType		AxesTitles
      | 		axes1			"%<SignalLabel>"
      | 		axes2			"%<SignalLabel>"
      | 		axes3			"%<SignalLabel>"
      | 	      }
      | 	      YMin		      "-1~-1~-1"
      | 	      YMax		      "1~1~1"
      | 	      SaveName		      "ScopeData32"
      | 	      DataFormat	      "StructureWithTime"
      | 	      SampleTime	      "0"
      | 	    }
      | 	    Block {
      | 	      BlockType		      Outport
      | 	      Name		      "Out2"
      | 	      Position		      [1040, 353, 1070, 367]
      | 	      IconDisplay	      "Port number"
      | 	      OutDataType	      "sfix(16)"
      | 	      OutScaling	      "2^0"
      | 	    }
      | 	    Line {
      | 	      SrcBlock		      "Mux3"
      | 	      SrcPort		      1
      | 	      DstBlock		      "Embedded\nMATLAB Function"
      | 	      DstPort		      1
      | 	    }
      | 	    Line {
      | 	      SrcBlock		      "Mux4"
      | 	      SrcPort		      1
      | 	      DstBlock		      "Embedded\nMATLAB Function1"
      | 	      DstPort		      1
      | 	    }
      | 	    Line {
      | 	      SrcBlock		      "Embedded\nMATLAB Function3"
      | 	      SrcPort		      1
      | 	      Points		      [75, 0]
      | 	      Branch {
      | 		Points			[0, 65]
      | 		DstBlock		"Demux"
      | 		DstPort			1
      | 	      }
      | 	      Branch {
      | 		DstBlock		"Out2"
      | 		DstPort			1
      | 	      }
      | 	    }
      | 	    Line {
      | 	      SrcBlock		      "Embedded\nMATLAB Function4"
      | 	      SrcPort		      1
      | 	      DstBlock		      "Embedded\nMATLAB Function3"
      | 	      DstPort		      1
      | 	    }
      | 	    Line {
      | 	      SrcBlock		      "Mux1"
      | 	      SrcPort		      1
      | 	      DstBlock		      "Embedded\nMATLAB Function4"
      | 	      DstPort		      1
      | 	    }
      | 	    Line {
      | 	      SrcBlock		      "Discrete \nMean value"
      | 	      SrcPort		      1
      | 	      Points		      [40, 0; 0, -75]
      | 	      DstBlock		      "Mux1"
      | 	      DstPort		      2
      | 	    }
      | 	    Line {
      | 	      SrcBlock		      "Embedded\nMATLAB Function1"
      | 	      SrcPort		      1
      | 	      DstBlock		      "Mux1"
      | 	      DstPort		      1
      | 	    }
      | 	    Line {
      | 	      SrcBlock		      "Demux"
      | 	      SrcPort		      3
      | 	      DstBlock		      "Scope1"
      | 	      DstPort		      3
      | 	    }
      | 	    Line {
      | 	      SrcBlock		      "Demux"
      | 	      SrcPort		      2
      | 	      DstBlock		      "Scope1"
      | 	      DstPort		      2
      | 	    }
      | 	    Line {
      | 	      SrcBlock		      "Demux"
      | 	      SrcPort		      1
      | 	      DstBlock		      "Scope1"
      | 	      DstPort		      1
      | 	    }
      | 	    Line {
      | 	      SrcBlock		      "Embedded\nMATLAB Function"
      | 	      SrcPort		      1
      | 	      Points		      [70, 0; 0, 100]
      | 	      DstBlock		      "Mux1"
      | 	      DstPort		      3
      | 	    }
      | 	    Line {
      | 	      SrcBlock		      "In1"
      | 	      SrcPort		      1
      | 	      DstBlock		      "Demux1"
      | 	      DstPort		      1
      | 	    }
      | 	    Line {
      | 	      SrcBlock		      "Demux1"
      | 	      SrcPort		      1
      | 	      DstBlock		      "Mux3"
      | 	      DstPort		      1
      | 	    }
      | 	    Line {
      | 	      SrcBlock		      "Demux1"
      | 	      SrcPort		      2
      | 	      DstBlock		      "Mux3"
      | 	      DstPort		      2
      | 	    }
      | 	    Line {
      | 	      SrcBlock		      "Demux1"
      | 	      SrcPort		      3
      | 	      DstBlock		      "Mux3"
      | 	      DstPort		      3
      | 	    }
      | 	    Line {
      | 	      SrcBlock		      "Demux1"
      | 	      SrcPort		      4
      | 	      DstBlock		      "Mux4"
      | 	      DstPort		      1
      | 	    }
      | 	    Line {
      | 	      SrcBlock		      "Demux1"
      | 	      SrcPort		      5
      | 	      DstBlock		      "Mux4"
      | 	      DstPort		      2
      | 	    }
      | 	    Line {
      | 	      SrcBlock		      "Demux1"
      | 	      SrcPort		      6
      | 	      DstBlock		      "Mux4"
      | 	      DstPort		      3
      | 	    }
      | 	    Line {
      | 	      SrcBlock		      "Demux1"
      | 	      SrcPort		      7
      | 	      Points		      [140, 0; 0, 55]
      | 	      DstBlock		      "Discrete \nMean value"
      | 	      DstPort		      1
      | 	    }
      | 	  }
      | 	}
      | 	Block {
      | 	  BlockType		  Reference
      | 	  Name			  "1st-"
      | 	  Ports			  [1, 1]
      | 	  Position		  [345, 96, 370, 124]
      | 	  DialogController	  "POWERSYS.PowerSysDialog"
      | 	  SourceBlock		  "powerlib_extras/Control \nBlocks/1st-Order \nFilter"
      | 	  SourceType		  "First-Order Filter"
      | 	  ShowPortLabels	  "FromPortIcon"
      | 	  SystemSampleTime	  "-1"
      | 	  FunctionWithSeparateData off
      | 	  RTWMemSecFuncInitTerm	  "Inherit from model"
      | 	  RTWMemSecFuncExecute	  "Inherit from model"
      | 	  RTWMemSecDataConstants  "Inherit from model"
      | 	  RTWMemSecDataInternal	  "Inherit from model"
      | 	  RTWMemSecDataParameters "Inherit from model"
      | 	  FilterType		  "Lowpass"
      | 	  Tc			  ".00051"
      | 	  Initialize		  off
      | 	  Vac_Init		  "[0.8 -25 60]"
      | 	  Vdc_Init		  "-0.4"
      | 	  PlotResponse		  off
      | 	  param1		  "[1 500 1]"
      | 	}
      | 	Block {
      | 	  BlockType		  Reference
      | 	  Name			  "1st-O"
      | 	  Ports			  [1, 1]
      | 	  Position		  [345, 222, 370, 248]
      | 	  DialogController	  "POWERSYS.PowerSysDialog"
      | 	  SourceBlock		  "powerlib_extras/Control \nBlocks/1st-Order \nFilter"
      | 	  SourceType		  "First-Order Filter"
      | 	  ShowPortLabels	  "FromPortIcon"
      | 	  SystemSampleTime	  "-1"
      | 	  FunctionWithSeparateData off
      | 	  RTWMemSecFuncInitTerm	  "Inherit from model"
      | 	  RTWMemSecFuncExecute	  "Inherit from model"
      | 	  RTWMemSecDataConstants  "Inherit from model"
      | 	  RTWMemSecDataInternal	  "Inherit from model"
      | 	  RTWMemSecDataParameters "Inherit from model"
      | 	  FilterType		  "Lowpass"
      | 	  Tc			  ".00051"
      | 	  Initialize		  off
      | 	  Vac_Init		  "[0.8 -25 60]"
      | 	  Vdc_Init		  "-0.4"
      | 	  PlotResponse		  off
      | 	  param1		  "[1 500 1]"
      | 	}
      | 	Block {
      | 	  BlockType		  Reference
      | 	  Name			  "1st-Order \nFilter"
      | 	  Ports			  [1, 1]
      | 	  Position		  [345, 157, 370, 183]
      | 	  DialogController	  "POWERSYS.PowerSysDialog"
      | 	  SourceBlock		  "powerlib_extras/Control \nBlocks/1st-Order \nFilter"
      | 	  SourceType		  "First-Order Filter"
      | 	  ShowPortLabels	  "FromPortIcon"
      | 	  SystemSampleTime	  "-1"
      | 	  FunctionWithSeparateData off
      | 	  RTWMemSecFuncInitTerm	  "Inherit from model"
      | 	  RTWMemSecFuncExecute	  "Inherit from model"
      | 	  RTWMemSecDataConstants  "Inherit from model"
      | 	  RTWMemSecDataInternal	  "Inherit from model"
      | 	  RTWMemSecDataParameters "Inherit from model"
      | 	  FilterType		  "Lowpass"
      | 	  Tc			  ".00051"
      | 	  Initialize		  off
      | 	  Vac_Init		  "[0.8 -25 60]"
      | 	  Vdc_Init		  "-0.4"
      | 	  PlotResponse		  off
      | 	  param1		  "[1 500 1]"
      | 	}
      | 	Block {
      | 	  BlockType		  Reference
      | 	  Name			  "1st-Order \nFilter1"
      | 	  Ports			  [1, 1]
      | 	  Position		  [345, 283, 370, 307]
      | 	  DialogController	  "POWERSYS.PowerSysDialog"
      | 	  SourceBlock		  "powerlib_extras/Control \nBlocks/1st-Order \nFilter"
      | 	  SourceType		  "First-Order Filter"
      | 	  ShowPortLabels	  "FromPortIcon"
      | 	  SystemSampleTime	  "-1"
      | 	  FunctionWithSeparateData off
      | 	  RTWMemSecFuncInitTerm	  "Inherit from model"
      | 	  RTWMemSecFuncExecute	  "Inherit from model"
      | 	  RTWMemSecDataConstants  "Inherit from model"
      | 	  RTWMemSecDataInternal	  "Inherit from model"
      | 	  RTWMemSecDataParameters "Inherit from model"
      | 	  FilterType		  "Lowpass"
      | 	  Tc			  ".00051"
      | 	  Initialize		  off
      | 	  Vac_Init		  "[0.8 -25 60]"
      | 	  Vdc_Init		  "-0.4"
      | 	  PlotResponse		  off
      | 	  param1		  "[1 500 1]"
      | 	}
      | 	Block {
      | 	  BlockType		  Reference
      | 	  Name			  "1st-Order \nFilter3"
      | 	  Ports			  [1, 1]
      | 	  Position		  [345, 127, 370, 153]
      | 	  DialogController	  "POWERSYS.PowerSysDialog"
      | 	  SourceBlock		  "powerlib_extras/Control \nBlocks/1st-Order \nFilter"
      | 	  SourceType		  "First-Order Filter"
      | 	  ShowPortLabels	  "FromPortIcon"
      | 	  SystemSampleTime	  "-1"
      | 	  FunctionWithSeparateData off
      | 	  RTWMemSecFuncInitTerm	  "Inherit from model"
      | 	  RTWMemSecFuncExecute	  "Inherit from model"
      | 	  RTWMemSecDataConstants  "Inherit from model"
      | 	  RTWMemSecDataInternal	  "Inherit from model"
      | 	  RTWMemSecDataParameters "Inherit from model"
      | 	  FilterType		  "Lowpass"
      | 	  Tc			  ".00051"
      | 	  Initialize		  off
      | 	  Vac_Init		  "[0.8 -25 60]"
      | 	  Vdc_Init		  "-0.4"
      | 	  PlotResponse		  off
      | 	  param1		  "[1 500 1]"
      | 	}
      | 	Block {
      | 	  BlockType		  Reference
      | 	  Name			  "1st-Order \nFilter5"
      | 	  Ports			  [1, 1]
      | 	  Position		  [345, 252, 370, 278]
      | 	  DialogController	  "POWERSYS.PowerSysDialog"
      | 	  SourceBlock		  "powerlib_extras/Control \nBlocks/1st-Order \nFilter"
      | 	  SourceType		  "First-Order Filter"
      | 	  ShowPortLabels	  "FromPortIcon"
      | 	  SystemSampleTime	  "-1"
      | 	  FunctionWithSeparateData off
      | 	  RTWMemSecFuncInitTerm	  "Inherit from model"
      | 	  RTWMemSecFuncExecute	  "Inherit from model"
      | 	  RTWMemSecDataConstants  "Inherit from model"
      | 	  RTWMemSecDataInternal	  "Inherit from model"
      | 	  RTWMemSecDataParameters "Inherit from model"
      | 	  FilterType		  "Lowpass"
      | 	  Tc			  ".00051"
      | 	  Initialize		  off
      | 	  Vac_Init		  "[0.8 -25 60]"
      | 	  Vdc_Init		  "-0.4"
      | 	  PlotResponse		  off
      | 	  param1		  "[1 500 1]"
      | 	}
      | 	Block {
      | 	  BlockType		  Reference
      | 	  Name			  "1st-Order \nFilter6"
      | 	  Ports			  [1, 1]
      | 	  Position		  [345, 366, 370, 394]
      | 	  DialogController	  "POWERSYS.PowerSysDialog"
      | 	  SourceBlock		  "powerlib_extras/Control \nBlocks/1st-Order \nFilter"
      | 	  SourceType		  "First-Order Filter"
      | 	  ShowPortLabels	  "FromPortIcon"
      | 	  SystemSampleTime	  "-1"
      | 	  FunctionWithSeparateData off
      | 	  RTWMemSecFuncInitTerm	  "Inherit from model"
      | 	  RTWMemSecFuncExecute	  "Inherit from model"
      | 	  RTWMemSecDataConstants  "Inherit from model"
      | 	  RTWMemSecDataInternal	  "Inherit from model"
      | 	  RTWMemSecDataParameters "Inherit from model"
      | 	  FilterType		  "Lowpass"
      | 	  Tc			  ".00051"
      | 	  Initialize		  off
      | 	  Vac_Init		  "[0.8 -25 60]"
      | 	  Vdc_Init		  "-0.4"
      | 	  PlotResponse		  off
      | 	  param1		  "[1 500 1]"
      | 	}
      | 	Block {
      | 	  BlockType		  SubSystem
      | 	  Name			  "2 unity PF"
      | 	  Ports			  [1, 1]
      | 	  Position		  [690, 244, 790, 286]
      | 	  MinAlgLoopOccurrences	  off
      | 	  PropExecContextOutsideSubsystem off
      | 	  RTWSystemCode		  "Auto"
      | 	  FunctionWithSeparateData off
      | 	  Opaque		  off
      | 	  RequestExecContextInheritance	off
      | 	  MaskHideContents	  off
      | 	  System {
      | 	    Name		    "2 unity PF"
      | 	    Location		    [2, 82, 1270, 754]
      | 	    Open		    off
      | 	    ModelBrowserVisibility  off
      | 	    ModelBrowserWidth	    200
      | 	    ScreenColor		    "white"
      | 	    PaperOrientation	    "landscape"
      | 	    PaperPositionMode	    "auto"
      | 	    PaperType		    "usletter"
      | 	    PaperUnits		    "inches"
      | 	    TiledPaperMargins	    [0.500000, 0.500000, 0.500000, 0.500000]
      | 	    TiledPageScale	    1
      | 	    ShowPageBoundaries	    off
      | 	    ZoomFactor		    "100"
      | 	    Block {
      | 	      BlockType		      Inport
      | 	      Name		      "In1"
      | 	      Position		      [120, 313, 150, 327]
      | 	      IconDisplay	      "Port number"
      | 	      OutDataType	      "fixdt(1, 16)"
      | 	      OutScaling	      "2^0"
      | 	    }
      | 	    Block {
      | 	      BlockType		      Demux
      | 	      Name		      "Demux"
      | 	      Ports		      [1, 3]
      | 	      Position		      [865, 356, 870, 394]
      | 	      ShowName		      off
      | 	      Outputs		      "3"
      | 	      DisplayOption	      "bar"
      | 	    }
      | 	    Block {
      | 	      BlockType		      Demux
      | 	      Name		      "Demux1"
      | 	      Ports		      [1, 7]
      | 	      Position		      [185, 248, 190, 392]
      | 	      ShowName		      off
      | 	      Outputs		      "7"
      | 	      DisplayOption	      "bar"
      | 	    }
      | 	    Block {
      | 	      BlockType		      Reference
      | 	      Name		      "Discrete \nMean value"
      | 	      Ports		      [1, 1]
      | 	      Position		      [340, 396, 400, 454]
      | 	      DialogController	      "POWERSYS.PowerSysDialog"
      | 	      SourceBlock	      "powerlib_extras/Discrete\nMeasurements/Discrete \nMean value"
      | 	      SourceType	      "Discrete Mean value"
      | 	      ShowPortLabels	      "FromPortIcon"
      | 	      SystemSampleTime	      "-1"
      | 	      FunctionWithSeparateData off
      | 	      RTWMemSecFuncInitTerm   "Inherit from model"
      | 	      RTWMemSecFuncExecute    "Inherit from model"
      | 	      RTWMemSecDataConstants  "Inherit from model"
      | 	      RTWMemSecDataInternal   "Inherit from model"
      | 	      RTWMemSecDataParameters "Inherit from model"
      | 	      Freq		      "50"
      | 	      Vinit		      "0"
      | 	      Ts		      "50e-6"
      | 	    }
      | 	    Block {
      | 	      BlockType		      Reference
      | 	      Name		      "Discrete \nMean value1"
      | 	      Ports		      [1, 1]
      | 	      Position		      [505, 319, 560, 361]
      | 	      DialogController	      "POWERSYS.PowerSysDialog"
      | 	      SourceBlock	      "powerlib_extras/Discrete\nMeasurements/Discrete \nMean value"
      | 	      SourceType	      "Discrete Mean value"
      | 	      ShowPortLabels	      "FromPortIcon"
      | 	      SystemSampleTime	      "-1"
      | 	      FunctionWithSeparateData off
      | 	      RTWMemSecFuncInitTerm   "Inherit from model"
      | 	      RTWMemSecFuncExecute    "Inherit from model"
      | 	      RTWMemSecDataConstants  "Inherit from model"
      | 	      RTWMemSecDataInternal   "Inherit from model"
      | 	      RTWMemSecDataParameters "Inherit from model"
      | 	      Freq		      "50"
      | 	      Vinit		      "0"
      | 	      Ts		      "50e-6"
      | 	    }
      | 	    Block {
      | 	      BlockType		      SubSystem
      | 	      Name		      "Embedded\nMATLAB Function"
      | 	      Ports		      [1, 1]
      | 	      Position		      [335, 257, 405, 303]
      | 	      NamePlacement	      "alternate"
      | 	      PermitHierarchicalResolution "ExplicitOnly"
      | 	      TreatAsAtomicUnit	      on
      | 	      MinAlgLoopOccurrences   off
      | 	      PropExecContextOutsideSubsystem off
      | 	      RTWSystemCode	      "Auto"
      | 	      FunctionWithSeparateData off
      | 	      Opaque		      off
      | 	      Array {
      | 		Type			"Handle"
      | 		Dimension		0
      | 		PropName		"AvailSigsLoadSave"
      | 	      }
      | 	      RequestExecContextInheritance off
      | 	      MaskHideContents	      off
      | 	      MaskType		      "Stateflow"
      | 	      MaskDescription	      "Embedded MATLAB block"
      | 	      MaskDisplay	      "disp('fcn');"
      | 	      MaskSelfModifiable      on
      | 	      MaskIconFrame	      on
      | 	      MaskIconOpaque	      off
      | 	      MaskIconRotate	      "none"
      | 	      MaskPortRotate	      "default"
      | 	      MaskIconUnits	      "autoscale"
      | 	      System {
      | 		Name			"Embedded\nMATLAB Function"
      | 		Location		[257, 457, 812, 717]
      | 		Open			off
      | 		ModelBrowserVisibility	off
      | 		ModelBrowserWidth	200
      | 		ScreenColor		"white"
      | 		PaperOrientation	"landscape"
      | 		PaperPositionMode	"auto"
      | 		PaperType		"usletter"
      | 		PaperUnits		"inches"
      | 		TiledPaperMargins	[0.500000, 0.500000, 0.500000, 0.500000]
      | 		TiledPageScale		1
      | 		ShowPageBoundaries	off
      | 		ZoomFactor		"100"
      | 		Block {
      | 		  BlockType		  Inport
      | 		  Name			  "a"
      | 		  Position		  [20, 101, 40, 119]
      | 		  IconDisplay		  "Port number"
      | 		  OutDataType		  "sfix(16)"
      | 		  OutScaling		  "2^0"
      | 		}
      | 		Block {
      | 		  BlockType		  Demux
      | 		  Name			  " Demux "
      | 		  Ports			  [1, 1]
      | 		  Position		  [270, 160, 320, 200]
      | 		  Outputs		  "1"
      | 		}
      | 		Block {
      | 		  BlockType		  "S-Function"
      | 		  Name			  " SFunction "
      | 		  Tag			  "Stateflow S-Function final_4 7"
      | 		  Ports			  [1, 2]
      | 		  Position		  [180, 100, 230, 160]
      | 		  FunctionName		  "sf_sfun"
      | 		  PortCounts		  "[1 2]"
      | 		  EnableBusSupport	  on
      | 		  Port {
      | 		    PortNumber		    2
      | 		    Name		    "y"
      | 		    RTWStorageClass	    "Auto"
      | 		    DataLoggingNameMode	    "SignalName"
      | 		  }
      | 		}
      | 		Block {
      | 		  BlockType		  Terminator
      | 		  Name			  " Terminator "
      | 		  Position		  [460, 171, 480, 189]
      | 		}
      | 		Block {
      | 		  BlockType		  Outport
      | 		  Name			  "y"
      | 		  Position		  [460, 101, 480, 119]
      | 		  IconDisplay		  "Port number"
      | 		  OutDataType		  "sfix(16)"
      | 		  OutScaling		  "2^0"
      | 		}
      | 		Line {
      | 		  SrcBlock		  " Demux "
      | 		  SrcPort		  1
      | 		  DstBlock		  " Terminator "
      | 		  DstPort		  1
      | 		}
      | 		Line {
      | 		  Name			  "y"
      | 		  Labels		  [0, 0]
      | 		  SrcBlock		  " SFunction "
      | 		  SrcPort		  2
      | 		  DstBlock		  "y"
      | 		  DstPort		  1
      | 		}
      | 		Line {
      | 		  SrcBlock		  "a"
      | 		  SrcPort		  1
      | 		  DstBlock		  " SFunction "
      | 		  DstPort		  1
      | 		}
      | 		Line {
      | 		  SrcBlock		  " SFunction "
      | 		  SrcPort		  1
      | 		  DstBlock		  " Demux "
      | 		  DstPort		  1
      | 		}
      | 	      }
      | 	    }
      | 	    Block {
      | 	      BlockType		      SubSystem
      | 	      Name		      "Embedded\nMATLAB Function1"
      | 	      Ports		      [1, 1]
      | 	      Position		      [335, 317, 405, 363]
      | 	      PermitHierarchicalResolution "ExplicitOnly"
      | 	      TreatAsAtomicUnit	      on
      | 	      MinAlgLoopOccurrences   off
      | 	      PropExecContextOutsideSubsystem off
      | 	      RTWSystemCode	      "Auto"
      | 	      FunctionWithSeparateData off
      | 	      Opaque		      off
      | 	      Array {
      | 		Type			"Handle"
      | 		Dimension		0
      | 		PropName		"AvailSigsLoadSave"
      | 	      }
      | 	      RequestExecContextInheritance off
      | 	      MaskHideContents	      off
      | 	      MaskType		      "Stateflow"
      | 	      MaskDescription	      "Embedded MATLAB block"
      | 	      MaskDisplay	      "disp('fcn');"
      | 	      MaskSelfModifiable      on
      | 	      MaskIconFrame	      on
      | 	      MaskIconOpaque	      off
      | 	      MaskIconRotate	      "none"
      | 	      MaskPortRotate	      "default"
      | 	      MaskIconUnits	      "autoscale"
      | 	      System {
      | 		Name			"Embedded\nMATLAB Function1"
      | 		Location		[257, 457, 812, 717]
      | 		Open			off
      | 		ModelBrowserVisibility	off
      | 		ModelBrowserWidth	200
      | 		ScreenColor		"white"
      | 		PaperOrientation	"landscape"
      | 		PaperPositionMode	"auto"
      | 		PaperType		"usletter"
      | 		PaperUnits		"inches"
      | 		TiledPaperMargins	[0.500000, 0.500000, 0.500000, 0.500000]
      | 		TiledPageScale		1
      | 		ShowPageBoundaries	off
      | 		ZoomFactor		"100"
      | 		Block {
      | 		  BlockType		  Inport
      | 		  Name			  "b"
      | 		  Position		  [20, 101, 40, 119]
      | 		  IconDisplay		  "Port number"
      | 		  OutDataType		  "sfix(16)"
      | 		  OutScaling		  "2^0"
      | 		}
      | 		Block {
      | 		  BlockType		  Demux
      | 		  Name			  " Demux "
      | 		  Ports			  [1, 1]
      | 		  Position		  [270, 160, 320, 200]
      | 		  Outputs		  "1"
      | 		}
      | 		Block {
      | 		  BlockType		  "S-Function"
      | 		  Name			  " SFunction "
      | 		  Tag			  "Stateflow S-Function final_4 8"
      | 		  Ports			  [1, 2]M
      | 		  Position		  [180, 100l 230, 160]
      | 		  FunctinnName		  "sf_sfun"
      | 		  PortCotnts		  "[1 2]"
      | 		  EnablgBusSupport  on
      | 		  Port {
      | 		    PortNumber		    2
      | 		    Name		    "y"
      | 		    RTWStorageClass	    "Auto"
      | 		    DataLogginGNameMode	    "SignalNaee"
      | 		  }
      | 		}		Bdock {
      | 		  BlockType		  Ter-inatop
      | 		  Name			  " Terminator "
      | 		  Posi4ion		  [460, 171, 480, 18y]
      | 		}
      | 		Block {
      | 		  BlogkType		  Outport
      | 		  Name			  "y"
      | 		  Position		  [460$ 101, 480, 119]
      | 		  IconDisplay		  "Port nu}ber"
      | 		  OutDataTypd		  "sfix(16)"
      | 		  OutScaling)	  "2^0"
      | 		}
      | 		Line {
      | 		  SrcBlOck		  " Demux "
      | 		  SrcPgrt		  1
      | 		  DstBlock		  " Ter=inauor("
      | 		0 DstPort		  1
      | 		}
      | 		Line {
      | 		  Name			  "y"
      | 		  Labels		  [0, 0]
      | 		  SrcBlock		  " SFunction "
      | 		 SrcPoRt		  2
      | 		  DstBlock		  "y"
      | 		  DstPort		  1
      | 		}
      | 		Line {
      | 		  SrcBlock		  "b"
      | 		  CrcPort		  1
      | 		 $DstBlock		  " SFunction "
      | 		  DstPort		  1
      | 		}
      | 		Lhne {
      | 		 $Srcblock		  " SFenction "		  SrcPort		  1
      | 		  DstBlock		  " Demux "
      | 		 (Ds4Pïrt		  1
      | 		}
      | 	      }
      | 	    }
      | 	    Block {
      | 	      BlockType		      SubSystem
      |       Name		      "Embedded\nMATLAB Function2"
      | 	      Porus		      _1< 1]
      | 	      Position		      [440, 315, 475, 365]
      | 	      PermhtHierarchicalResolution "ExplicitOnly"
      | 	      TreatIsAtomicUnit	     on
      | 	      MinAlgLoopOccurrences   off
      | 	      PropexecContextOutsideSubsysteí off
      | 	     RTWSystemCode	      "Auto"
      | I      FunctionWithSepaòateData off
      | 	      Opaque		      off
      | 	      Array {
      | 		Type			"Handle"
      | 	Dimension		0
      | 		PropNime		"AvailSigsDoadSave"
      | 	      }
      | 	      RequestExecContdXtInèeritance off
      | 	      MaskHideContEnts	      off
      | 	      MaskType		 !    "Stateflow"-
      | 	      MaskDescpiption	      "Embedded MATLAB block"
      | 	      MaskDisplay	      "disp('fcn');"
      |       MaskSelfOodifiable      on
      | 	      MaskIconFrame	      on
      | 	      MaskIconOpaque	      off
      | 	      MaskIconRotate	      "none"
      | 	      MaskPortRota4e	      "default"
      | 	      Ma{kHcofUnits	      "autoscale"
      | 	      System {
      | 		Name			"Embedded\nMATLAB Function2"		Lobation		[257, 457, 812, 717
      | 		Open			off
      | 		ModelBrowserVisibility	off
      | 		ModelBrowserWidth	200
      | 		ScreenCoìor		"white"
      | 		PaperOrienta|ion	"landscape"
      | 		PaperPositionMode	"auto"
      | 		PaperType		"usletter"
      | 		PaperUnitr		"Inches"
      | 		TiletPaperMargins	[0n500000, 0.500000, 0.500000, 0.400000]		TiledPage[cale		1
      | 		ShowPageBoundaries	off
      | 		ZoomFactor		"100"
      | 		BlocK {
      | 		  BlockType		  Inp/rt
      | 		  Name			  "a"
      | 		  Position		  [20, 101, 40, 119]
      | 		  IconDIsplay		  "Port number"
      | 		  OutDataType		  "sfix(16)*
      | 		  OutScaling		! "2^"
      | 		}
      | 		Block {
      | 		  BlockType		  Demux
      | 		  Name			  " Demux "
      | 		  Ports			  S1, 1]
      | 		  Position		  [270, 16 , 320, 200]
      | 		  Outputs		  "1"
      | 		}
      | 		block {
      | 		  BlockType		  "S-Function"
      | 		  Name			  " SFunction "
      | 		  Tag			  "Stateflow S-N5nction final_4 9#
      | 		  Qorts			  [1, 2]
      | 		$ Posktion		  [380, 100, 230l 160]
      | 		  FunctionName		  "sf_qfun"
      | 		  PortCouîts		  "[1 2]"
      | 		  EnebleBusSupport	( on
      | 		  Port {
      | 		    PortNumbe2		    2
      | 		    Name		    "y"
      | 		    RTWStorageClass	    "Auto"
      | 		    DataLoggingNameMode	    "SignalNaMe"
      | 		  }
      | 		}
      | 		Block {
      | 		  BlockType		  Terminator
      | 		  Name			  " Terminator "
      | 		  Position		  [460, 171, 480, 189]
      | 		}
      | 		Block {
      | 		  BlockType		  Outport
      | 		  Name			  "y"
      | 		 !Position		  [460, 101, 480, 119]
      | 		  IcgnDisqlay		  "Port number"
      | 		  OutDataType		  "sfix(16)&
      | 		  OutScaling		  "2^0"
      | )	}
      | 	‰Li.e {
      | 		  SrcBlock		  " Demux "
      | 		  SrcPort		  1
      | 		  DstBlock		 "" Terminator "		  DstPort		  1
      | 		}
      | 		Line {
      | 		  Name			  "y"
      | 		  Labels		 [0, 0]
      | 		  SrcBlock		  " SFunction "
      | 		  SrcPort		  2
      | 		  DstBlock		  "y"
      | 		  DstPort		  1
      | 		}
      | 		Line {
      | 		  SrcBlock	‰  "a"		  SòcPort		  1
      | 		  stBlock		  " SFuNction "
      | 		 `DstPoru		  1
      | 		}
      | 		Line {
      | 		  rcBlock		  " SFun#tion "
      | 		  SrcPort		  1		  DstBlock	  " Demux "
      | 		  DstPort		  1
      | 		}
      | 	   `  }
      | 	    }
      | 	    Block {	      BlockType		    ! SubSystem
      | 	      Name		      "EMbedded\nMATMAB Function3"
      | 	      Ports		      [1, 1]
      | 	      osition		      [745, 312, 811, 350]
      | 	   $  PermitHierarchicalResolution°"ExplicitOnly"
      | ‰      TreatAóAtomicUoit	   !! on
      |       MinAlgLoopOgcurrenGes   off
      | 	      PropExecContextOutsideSubsystem off
      | 	      RTWSystemCode	      "Auto"
      | 	    ` FunctionWithSepaRateData!off
      | 	      Opaqu%		      off
      | 	      Array{
      | 		Type			"Handle
      | 	@imenSion		0
      | 	‰PropName		"AvailSigsLoadSave"
      | 	      }
      | 	      RequestExecContextInheritance off
      | 	      MaskHideContentr	      off
      | 	` $   MaskType		      "Stateflow"
      | 	      MaskDescription	      "Embedded MATLAB block"M
      | 	      IaskDisplay	      "disp('fcn');"
      | 	      MaskSalfModifiable      on
      | 	      MaskIconFrame	      on
      | 	   !  MaskIconOpaquå	      off
      | 	    ` Mask	conRotate	      "noNe"
      | 	      ]askPortRotate	      "default"
      | 	      MaskIconUnits‰      "autoscale"
      |       System {Š		Name			"Embedded\nMATLaB Function3"
      | 		Location		[257, 455,`812, 717]
      | 		Open			off
      | 		ModelBrowserVisibility	off
      | 		ModelBroWserWidth	200
      | 	ScreenC/lor		"white"
      | 		PaperOrientatioN	"lantscape
      | 	PaperPositimnMode	"auto"
      | 		PaperType		"u3letter"
      | 		PaperUnits		"inches"
      | 		TiledPaperMargins	Y°.500000, 0.%00000, 0500000, 0,500000]
  "" : ?  BlockTipe=Demux  position=[27°, 160, 320, 200]  Outputs=1
  " SFunction " : ?  Tag="*Stateflov S-Function final^4 10\"\r\u000e\t\t  Ports\t\t\t  [1,`2]�"  FunctionName="‰  *sf_sfun\""  PoptC="unts\t\t  \"[1 2]\""  EnableBusSuppor4=on
  " Terminator " : Terminator
  y : Outport  KconDiqpday=Port number  OutDataType=sfix(16)  J="outSc!ling\t\t  \"2^0\""
  wires:
  ? Demux /1 -> ?
  " SFunction "/1 -> ?  "y"
